simulink model "Attitude_control_RW"  (R2021b)
settings: Solver=VariableStepAuto  StartTime=0.0  StopTime=200  FixedStep=0.0001  RelTol=1e-3
values from neighbouring files (symbols this model uses):
  R = 6378000 + h    (= 7078000)    [dynamicFunctions2.m]
  w0 = sqrt(mu_earth/(R^3))    [dynamicFunctions2.m]
undefined symbols (not defined in the file or in its folder): b, Is, kk, Km, Kt, Q, q_init, Rgyro, Rstr, rw_Inertia, rw_SensorToBody, Ts, unit7, w_dot_init, w_init, wRW_init
libraries: simulink_extras x10, sharedtransform x5, simulink x3, aerolibutil x1, sharedTrackingLibrary x1
settings Model: Creator=sokserey  LastModifiedBy=ASUS
settings SolverCC: ZeroCrossAlgorithm=Adaptive
settings DebuggingCC: IgnoredZcDiagnostic=none

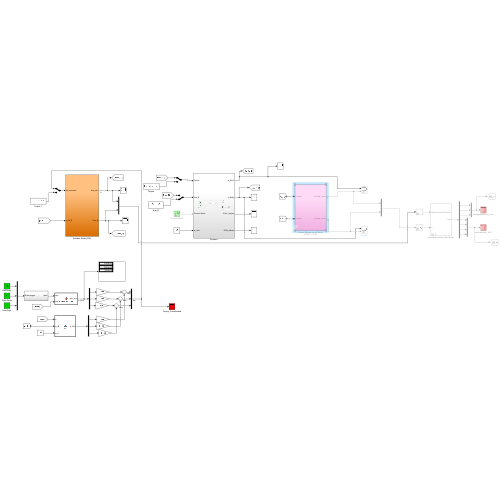
[thumbnail: Simulink's stored preview of the top-level diagram]
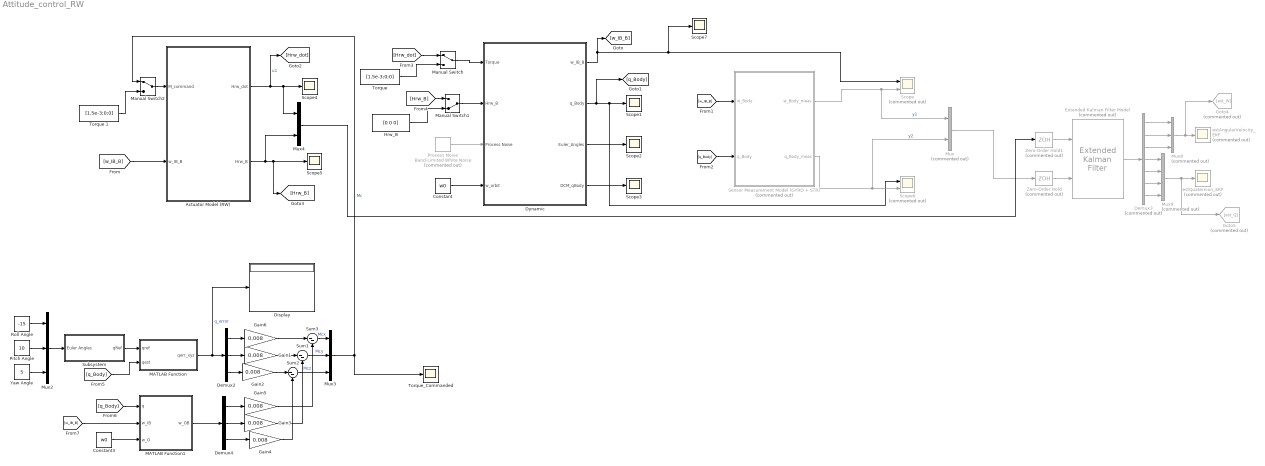
== system Attitude_control_RW ==
  Actuator Model (RW) : Subsystem
  Constant : Constant  Value=w0
  Constant3 : Constant  Value=w0
  Demux2 : Demux  Outputs=3
  Demux3 : Demux  Commented=on  Outputs=7
  Demux4 : Demux  Outputs=3
  Display : Display
  Dynamic : Subsystem
  "Extended Kalman Filter Model " : sharedTrackingLibrary/Extended Kalman Filter  Commented=on  StateTransitionFcn=dynamicFunctions2  HasStateTransitionJacobianFcn=off  HasAdditiveProcessNoise=Additive  ProcessNoise=diag(unit7)*Q  HasTimeVaryingProcessNoise=off  HasStateTransitionFcnExtraArgument=1  InitialState=[w_init; q_init]  InitialStateCovariance=1e-6  MeasurementFcn1=measurementFunction2  HasMeasurementJacobianFcn1=off  HasMeasurementEnablePort1=off  HasAdditiveMeasurementNoise1=Additive  MeasurementNoise1=Rconf4  HasTimeVaryingMeasurementNoise1=off  HasMeasurementFcnExtraArgument1=0  MeasurementFcn2=myMeasurementFcn  HasMeasurementJacobianFcn2=off  HasMeasurementEnablePort2=off  HasAdditiveMeasurementNoise2=Additive  MeasurementNoise2=1  HasTimeVaryingMeasurementNoise2=off  HasMeasurementFcnExtraArgument2=0  MeasurementFcn3=myMeasurementFcn  HasMeasurementJacobianFcn3=off  HasMeasurementEnablePort3=off  HasAdditiveMeasurementNoise3=Additive  MeasurementNoise3=1  HasTimeVaryingMeasurementNoise3=off  HasMeasurementFcnExtraArgument3=0  MeasurementFcn4=myMeasurementFcn  HasMeasurementJacobianFcn4=off  HasMeasurementEnablePort4=off  HasAdditiveMeasurementNoise4=Additive  MeasurementNoise4=1  HasTimeVaryingMeasurementNoise4=off  HasMeasurementFcnExtraArgument4=0  MeasurementFcn5=myMeasurementFcn  HasMeasurementJacobianFcn5=off  HasMeasurementEnablePort5=off  HasAdditiveMeasurementNoise5=Additive  MeasurementNoise5=1  HasTimeVaryingMeasurementNoise5=off  HasMeasurementFcnExtraArgument5=0  EnableMultirate=off  StateTransitionFcnSampleTime=1  MeasurementFcn1SampleTime=1  MeasurementFcn2SampleTime=1  MeasurementFcn3SampleTime=1  MeasurementFcn4SampleTime=1  MeasurementFcn5SampleTime=1  UseCurrentEstimator=on  OutputStateCovariance=off  DataType=double  SampleTime=Ts  NumberOfMeasurements=1
      settings: SourceProductBaseCode=AE,PW,CT,DR,TF,ID,LP,NV,AR,RO,RR,UV,VE
  Gain{1..6} (6 alike) : Gain  Gain=0.008
  Goto4 : Goto  Commented=on  GotoTag=est_W
  Goto5 : Goto  Commented=on  GotoTag=est_Q
  Hrw_B : Constant  Value=[0 0 0]
  MATLAB Function : MATLAB Function  TreatAsAtomicUnit=on
  MATLAB Function1 : MATLAB Function  TreatAsAtomicUnit=on
  Manual Switch : ManualSwitch
  Manual Switch1 : ManualSwitch  CurrentSetting=0
  Manual Switch2 : ManualSwitch
  Mux : Mux  Commented=on  Inputs=2
  Mux2 : Mux  Inputs=3
  Mux3 : Mux  Inputs=3
  Mux4 : Mux  Inputs=2
  Mux8 : Mux  Commented=on  Inputs=3
  Mux9 : Mux  Commented=on
  Pitch Angle : Constant  Value=10
  Process Noise : simulink/Sources/Band-Limited White Noise  Commented=on  Cov=Q*Ts  Ts=Ts  seed=[23341]
  Roll Angle : Constant  Value=-15
  Scope : Scope  Commented=on  NumInputPorts=2
  Scope{1..5,7} (6 alike) : Scope
  Scope6 : Scope  Commented=on  NumInputPorts=2
  Sensor Measurement Model (GYRO + STR) : Subsystem  Commented=on
  Subsystem : Subsystem
  Sum1 : Sum  Inputs=|--
  Sum2 : Sum  Inputs=|--
  Sum3 : Sum  Inputs=|--
  "Torque " : Constant  Value=[1.5e-3;0;0]
  Torque 1 : Constant  Value=[1.5e-3;0;0]
  Torque_Commanded : Scope
  Yaw Angle : Constant  Value=5
  Zero-Order Hold : ZeroOrderHold  Commented=on  SampleTime=Ts
  Zero-Order Hold1 : ZeroOrderHold  Commented=on  SampleTime=Ts
  estAngularVelocity_EKF : Scope  Commented=on
  "estQuaternion_EKF " : Scope  Commented=on
  wires:
  Process Noise/1 -> Dynamic/3("Process Noise ")
  Constant/1 -> Dynamic/4(w_orbit)
  Dynamic/1(w_IB_B) -> [w_IB_B], Scope7/1, Scope/1
  Dynamic/2(q_Body) -> [q_Body], Scope6/1, Scope1/1
  Dynamic/3(Euler_Angles) -> Scope2/1
  Dynamic/4(DCM_qBody) -> Scope3/1
  Zero-Order Hold1/1 -> "Extended Kalman Filter Model "/1
  Demux3/2 -> Mux8/2
  Demux3/3 -> Mux8/3
  Demux3/6 -> Mux9/3
  Demux3/4 -> Mux9/1
  Mux9/1 -> Goto5/1, "estQuaternion_EKF "/1
  Demux3/5 -> Mux9/2
  "Extended Kalman Filter Model "/1 -> Demux3/1
  Demux3/1 -> Mux8/1
  Zero-Order Hold/1 -> "Extended Kalman Filter Model "/2
  [w_IB_B] -> Actuator Model (RW)/2(w_IB_B)
  Actuator Model (RW)/1("Hrw_dot ") -> [Hrw_dot], Mux4/1, Scope4/1  "u1"
  Actuator Model (RW)/2(Hrw_B) -> Mux4/2, [Hrw_B], Scope5/1
  [w_IB_B] -> Sensor Measurement Model (GYRO + STR)/1(w_Body)
  Sensor Measurement Model (GYRO + STR)/1(w_Body_meas) -> Mux/1, Scope/2  "y1"
  [q_Body] -> Sensor Measurement Model (GYRO + STR)/2(q_Body)
  Sensor Measurement Model (GYRO + STR)/2(q_Body_meas) -> Mux/2, Scope6/2  "y2"
  Mux/1 -> Zero-Order Hold/1
  "Torque "/1 -> Manual Switch/2
  Manual Switch1/1 -> Dynamic/2(Hrw_B)
  Hrw_B/1 -> Manual Switch1/2
  [Hrw_dot] -> Manual Switch/1
  [Hrw_B] -> Manual Switch1/1
  Roll Angle/1 -> Mux2/1
  Sum1/1 -> Mux3/2  "Mcy"
  MATLAB Function/1(qerr_xyz) -> Display/1, Demux2/1  "q_error"
  Demux4/2 -> Gain3/1
  Sum3/1 -> Mux3/1  "Mcx"
  Gain2/1 -> Sum2/1
  Sum2/1 -> Mux3/3  "Mcz"
  Demux4/1 -> Gain5/1
  Demux2/2 -> Gain1/1
  Demux2/1 -> Gain6/1
  Gain6/1 -> Sum3/1
  Mux3/1 -> Manual Switch2/1, Torque_Commanded/1  "Mc"
  Yaw Angle/1 -> Mux2/3
  Subsystem/1(qRef) -> MATLAB Function/1(qref)
  Gain1/1 -> Sum1/1
  Pitch Angle/1 -> Mux2/2
  Mux2/1 -> Subsystem/1(Euler Angles)
  Demux2/3 -> Gain2/1
  Mux8/1 -> Goto4/1, estAngularVelocity_EKF/1
  Demux4/3 -> Gain4/1
  Manual Switch2/1 -> Actuator Model (RW)/1("M_command ")
  Torque 1/1 -> Manual Switch2/2
  Demux3/7 -> Mux9/4
  Mux4/1 -> Zero-Order Hold1/1
  [q_Body] -> MATLAB Function/2(qest)
  [q_Body] -> MATLAB Function1/1(q)
  [w_IB_B] -> MATLAB Function1/2(w_IB)
  Constant3/1 -> MATLAB Function1/3(w_O)
  MATLAB Function1/1(w_OB) -> Demux4/1
  Gain5/1 -> Sum3/2
  Gain3/1 -> Sum1/2
  Gain4/1 -> Sum2/2
  Manual Switch/1 -> Dynamic/1(Torque)

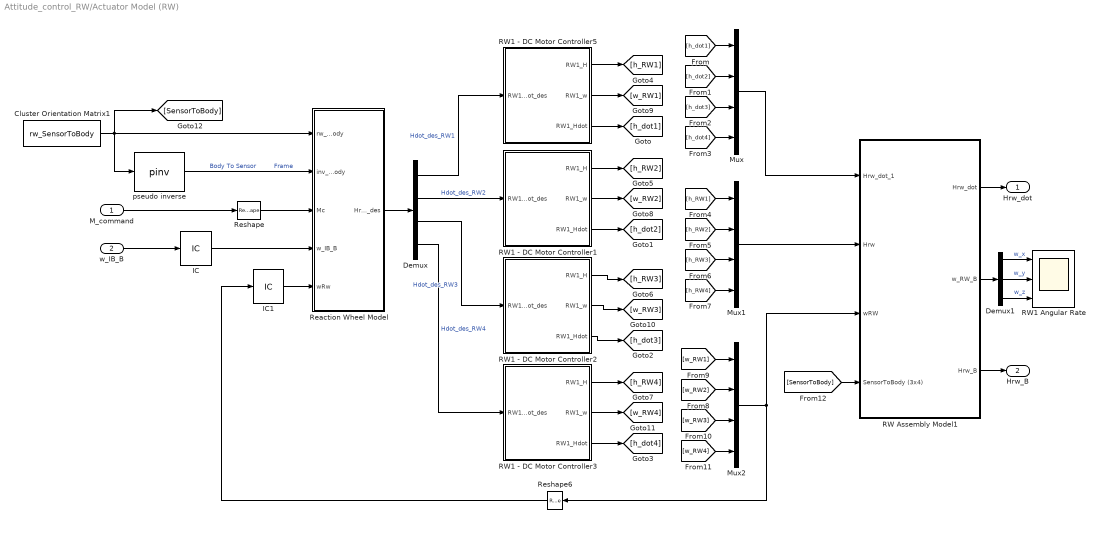
== system Attitude_control_RW/Actuator Model (RW) ==
  "M_command " : Inport
  w_IB_B : Inport  Port=2
  Cluster Orientation Matrix1 : Constant  Value=rw_SensorToBody  VectorParams1D=off  SampleTime=Ts
  Demux : Demux
  Demux1 : Demux  Outputs=3
  IC : InitialCondition  Value=w_init
  IC1 : InitialCondition  Value=wRW_init
  Mux : Mux
  Mux1 : Mux
  Mux2 : Mux
  RW Assembly Model1 : Subsystem
  RW1 - DC Motor Controller1 : Subsystem
  RW1 - DC Motor Controller2 : Subsystem
  RW1 - DC Motor Controller3 : Subsystem
  RW1 - DC Motor Controller5 : Subsystem
  RW1 Angular Rate : Scope  NumInputPorts=3
  Reaction Wheel Model : MATLAB Function  TreatAsAtomicUnit=on
  Reshape : Reshape  OutputDimensionality=Column vector (2-D)
  Reshape6 : Reshape  OutputDimensionality=Column vector (2-D)
  pseudo inverse : MATLABFcn  MATLABFcn=pinv  Output1D=off
  "Hrw_dot " : Outport  VectorParamsAs1DForOutWhenUnconnected=off
  Hrw_B : Outport  Port=2  VectorParamsAs1DForOutWhenUnconnected=off
  wires:
  Demux/1 -> RW1 - DC Motor Controller5/1(RW1_Hdot_des)  "Hdot_des_RW1"
  Demux/2 -> RW1 - DC Motor Controller1/1(RW1_Hdot_des)  "Hdot_des_RW2"
  Demux/3 -> RW1 - DC Motor Controller2/1(RW1_Hdot_des)  "Hdot_des_RW3"
  Demux/4 -> RW1 - DC Motor Controller3/1(RW1_Hdot_des)  "Hdot_des_RW4"
  Demux1/3 -> RW1 Angular Rate/3  "w_z"
  Demux1/1 -> RW1 Angular Rate/1  "w_x"
  Demux1/2 -> RW1 Angular Rate/2  "w_y"
  "M_command "/1 -> Reshape/1
  Reaction Wheel Model/1(Hrw_dot_des) -> Demux/1
  [h_dot1] -> Mux/1
  [h_dot2] -> Mux/2
  [h_dot3] -> Mux/3
  [h_dot4] -> Mux/4
  Mux/1 -> RW Assembly Model1/1(Hrw_dot_1)
  [h_RW1] -> Mux1/1
  [h_RW2] -> Mux1/2
  [h_RW3] -> Mux1/3
  [h_RW4] -> Mux1/4
  Mux1/1 -> RW Assembly Model1/2(Hrw)
  [w_RW2] -> Mux2/2
  [w_RW1] -> Mux2/1
  [w_RW3] -> Mux2/3
  [w_RW4] -> Mux2/4
  pseudo inverse/1 -> Reaction Wheel Model/2(inv_rwSensorToBody)  "Body To Sensor         Frame"
  Reshape/1 -> Reaction Wheel Model/3(Mc)
  Cluster Orientation Matrix1/1 -> pseudo inverse/1, [SensorToBody], Reaction Wheel Model/1(rw_SensorToBody)
  [SensorToBody] -> RW Assembly Model1/4(SensorToBody (3x4))
  RW Assembly Model1/2(w_RW_B) -> Demux1/1
  RW Assembly Model1/1(Hrw_dot) -> "Hrw_dot "/1
  Mux2/1 -> Reshape6/1, RW Assembly Model1/3(wRW)
  Reshape6/1 -> IC1/1
  w_IB_B/1 -> IC/1
  IC/1 -> Reaction Wheel Model/4(w_IB_B)
  IC1/1 -> Reaction Wheel Model/5(wRw)
  RW1 - DC Motor Controller5/2(RW1_w) -> [w_RW1]
  RW1 - DC Motor Controller5/1(RW1_H) -> [h_RW1]
  RW1 - DC Motor Controller5/3(RW1_Hdot) -> [h_dot1]
  RW1 - DC Motor Controller1/1(RW1_H) -> [h_RW2]
  RW1 - DC Motor Controller1/2(RW1_w) -> [w_RW2]
  RW1 - DC Motor Controller1/3(RW1_Hdot) -> [h_dot2]
  RW1 - DC Motor Controller2/1(RW1_H) -> [h_RW3]
  RW1 - DC Motor Controller2/2(RW1_w) -> [w_RW3]
  RW1 - DC Motor Controller2/3(RW1_Hdot) -> [h_dot3]
  RW1 - DC Motor Controller3/1(RW1_H) -> [h_RW4]
  RW1 - DC Motor Controller3/2(RW1_w) -> [w_RW4]
  RW1 - DC Motor Controller3/3(RW1_Hdot) -> [h_dot4]
  RW Assembly Model1/3(Hrw_B) -> Hrw_B/1

== system Attitude_control_RW/Dynamic ==
  Torque : Inport
  Hrw_B : Inport  Port=2
  "Process Noise " : Inport  Port=3
  w_orbit : Inport  Port=4
  Display2 : Display
  Dynamic Model : Subsystem
  Kinematic Model1 : Subsystem
  Subsystem : Subsystem
  Subsystem1 : Subsystem
  Sum1 : Sum  Inputs=|++
  Sum2 : Sum  Inputs=|++
  Terminator : Terminator
  w_IB_B : Outport  VectorParamsAs1DForOutWhenUnconnected=off
  q_Body : Outport  Port=2  VectorParamsAs1DForOutWhenUnconnected=off
  Euler_Angles : Outport  Port=3  VectorParamsAs1DForOutWhenUnconnected=off
  DCM_qBody : Outport  Port=4  VectorParamsAs1DForOutWhenUnconnected=off
  wires:
  Sum2/1 -> Dynamic Model/2("Hrw_B ")
  Dynamic Model/1(w_IB_B) -> Kinematic Model1/1(w_IB_B), w_IB_B/1
  Hrw_B/1 -> Sum2/1
  Sum1/1 -> Dynamic Model/1(Mc+Md)
  Subsystem1/1(Euler Angle) -> Euler_Angles/1
  Torque/1 -> Sum1/1
  Kinematic Model1/2(w_OB_B) -> Terminator/1
  Kinematic Model1/1(qBody) -> Subsystem/1(qest), q_Body/1
  "Process Noise "/1 -> Sum2/2, Sum1/2
  Subsystem/1("DCM ") -> Display2/1, DCM_qBody/1, Subsystem1/1("DCM ")
  w_orbit/1 -> Kinematic Model1/2(w_orbit)

== system Attitude_control_RW/Sensor Measurement Model (GYRO + STR) ==
  w_Body : Inport
  q_Body : Inport  Port=2
  GYRO Sensor Model : Subsystem
  Normalization Model : Subsystem
  Star Tracker Model : Subsystem
  w_Body_meas : Outport  VectorParamsAs1DForOutWhenUnconnected=off
  q_Body_meas : Outport  Port=2  VectorParamsAs1DForOutWhenUnconnected=off
  wires:
  GYRO Sensor Model/1(w_Body_meas) -> w_Body_meas/1
  w_Body/1 -> GYRO Sensor Model/1(w_Body)
  q_Body/1 -> Star Tracker Model/1(q_Body)
  Normalization Model/1(Normalized_u) -> q_Body_meas/1
  Star Tracker Model/1(q_Body_meas) -> Normalization Model/1(u)

== system Attitude_control_RW/Subsystem ==
  Euler Angles : Inport
  Degrees to Radians1 : simulink_extras/Transformations/Degrees to Radians
  Direction Cosine Matrix to Quaternions : sharedtransform/Direction Cosine Matrix  to Quaternions  aMode=0  action=None  tolerance=eps(2)
      settings: SourceProductBaseCode=AE,PW,DR,MT,UV,VE
  Rotation Angles to Direction Cosine Matrix : sharedtransform/Rotation Angles to Direction Cosine Matrix  rotationOrder=ZYX  aMode=aMode
      settings: SourceProductBaseCode=AE,PW,DR,MT,UV,VE
  Subsystem1 : Subsystem
  qRef : Outport  VectorParamsAs1DForOutWhenUnconnected=off
  wires:
  Euler Angles/1 -> Degrees to Radians1/1
  Degrees to Radians1/1 -> Rotation Angles to Direction Cosine Matrix/1
  Rotation Angles to Direction Cosine Matrix/1 -> Direction Cosine Matrix to Quaternions/1
  Direction Cosine Matrix to Quaternions/1 -> Subsystem1/1(q0,q1,q2,q3)
  Subsystem1/1(q1,q2,q3,q4) -> qRef/1

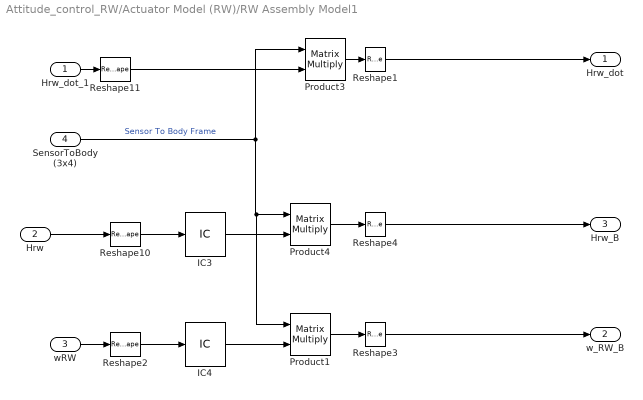
== system Attitude_control_RW/Actuator Model (RW)/RW Assembly Model1 ==
  Hrw_dot_1 : Inport
  Hrw : Inport  Port=2
  wRW : Inport  Port=3
  SensorToBody (3x4) : Inport  Port=4
  IC3 : InitialCondition  Value=[wRW_init(1,1)*rw_Inertia; wRW_init(2,1)*rw_Inertia; wRW_init(3,1)*rw_Inertia;wRW_init(4,1)*rw_Inertia]
  IC4 : InitialCondition  Value=wRW_init
  Product1 : Product  Inputs=**  Multiplication=Matrix(*)  RndMeth=Zero
  Product3 : Product  Inputs=**  Multiplication=Matrix(*)  RndMeth=Zero
  Product4 : Product  Inputs=**  Multiplication=Matrix(*)  RndMeth=Zero
  Reshape{1..4,10..11} (6 alike) : Reshape  OutputDimensionality=Column vector (2-D)
  Hrw_dot : Outport  VectorParamsAs1DForOutWhenUnconnected=off
  w_RW_B : Outport  Port=2  VectorParamsAs1DForOutWhenUnconnected=off
  Hrw_B : Outport  Port=3  VectorParamsAs1DForOutWhenUnconnected=off
  wires:
  SensorToBody (3x4)/1 -> Product3/1, Product1/1, Product4/1  "Sensor To Body Frame"
  Product4/1 -> Reshape4/1
  Reshape1/1 -> Hrw_dot/1
  Reshape4/1 -> Hrw_B/1
  IC3/1 -> Product4/2
  IC4/1 -> Product1/2
  Product1/1 -> Reshape3/1
  Hrw/1 -> Reshape10/1
  Reshape10/1 -> IC3/1
  Reshape2/1 -> IC4/1
  wRW/1 -> Reshape2/1
  Reshape3/1 -> w_RW_B/1
  Reshape11/1 -> Product3/2
  Hrw_dot_1/1 -> Reshape11/1
  Product3/1 -> Reshape1/1

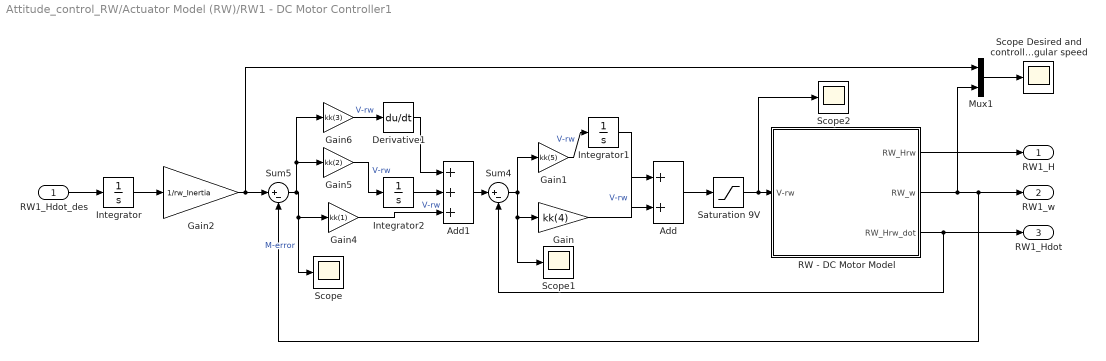
== system Attitude_control_RW/Actuator Model (RW)/RW1 - DC Motor Controller1 ==
  RW1_Hdot_des : Inport
  Add : Sum
  Add1 : Sum  Inputs=+++
  Derivative1 : Derivative
  Gain : Gain  Gain=kk(4)
  Gain1 : Gain  Gain=kk(5)
  Gain2 : Gain  Gain=1/rw_Inertia
  Gain4 : Gain  Gain=kk(1)
  Gain5 : Gain  Gain=kk(2)
  Gain6 : Gain  Gain=kk(3)
  Integrator : Integrator
  Integrator1 : Integrator
  Integrator2 : Integrator
  Mux1 : Mux  Inputs=2
  RW - DC Motor Model : Subsystem
  "Saturation 9V " : Saturate  UpperLimit=9  LowerLimit=-9
  Scope : Scope
  "Scope Desired and controlled RW-angular speed " : Scope
  Scope1 : Scope
  Scope2 : Scope
  Sum4 : Sum  Inputs=|+-
  Sum5 : Sum  Inputs=|+-
  RW1_H : Outport  VectorParamsAs1DForOutWhenUnconnected=off
  RW1_w : Outport  Port=2  VectorParamsAs1DForOutWhenUnconnected=off
  RW1_Hdot : Outport  Port=3  VectorParamsAs1DForOutWhenUnconnected=off
  wires:
  Gain4/1 -> Add1/3  "V-rw"
  Gain6/1 -> Derivative1/1  "V-rw"
  Derivative1/1 -> Add1/1
  RW - DC Motor Model/3(RW_Hrw_dot) -> Sum4/2, RW1_Hdot/1
  Add1/1 -> Sum4/1
  Gain1/1 -> Integrator1/1  "V-rw"
  "Saturation 9V "/1 -> Scope2/1, RW - DC Motor Model/1(V-rw)
  Add/1 -> "Saturation 9V "/1
  Integrator1/1 -> Add/2
  Sum5/1 -> Gain6/1, Gain5/1, Scope/1, Gain4/1  "M-error"
  Mux1/1 -> "Scope Desired and controlled RW-angular speed "/1
  Sum4/1 -> Gain/1, Scope1/1, Gain1/1
  RW - DC Motor Model/1(RW_Hrw) -> RW1_H/1
  Gain5/1 -> Integrator2/1  "V-rw"
  RW1_Hdot_des/1 -> Integrator/1
  RW - DC Motor Model/2(RW_w) -> Sum5/2, RW1_w/1, Mux1/2
  Integrator/1 -> Gain2/1
  Integrator2/1 -> Add1/2
  Gain2/1 -> Mux1/1, Sum5/1
  Gain/1 -> Add/1  "V-rw"

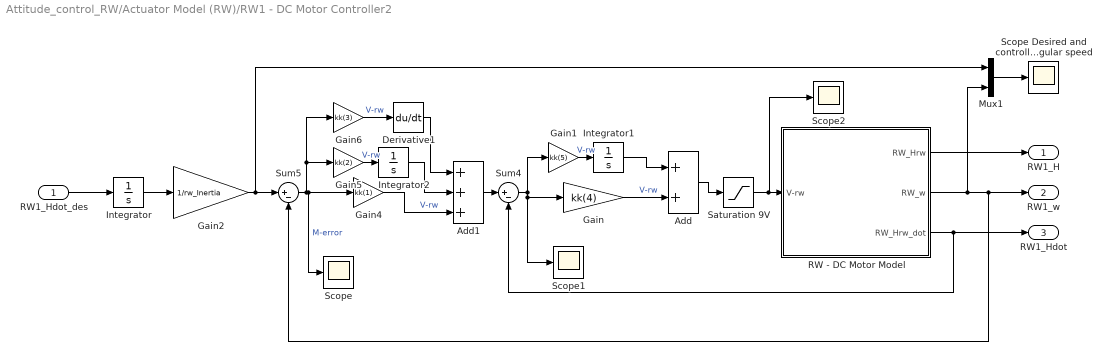
== system Attitude_control_RW/Actuator Model (RW)/RW1 - DC Motor Controller2 ==
  RW1_Hdot_des : Inport
  Add : Sum
  Add1 : Sum  Inputs=+++
  Derivative1 : Derivative
  Gain : Gain  Gain=kk(4)
  Gain1 : Gain  Gain=kk(5)
  Gain2 : Gain  Gain=1/rw_Inertia
  Gain4 : Gain  Gain=kk(1)
  Gain5 : Gain  Gain=kk(2)
  Gain6 : Gain  Gain=kk(3)
  Integrator : Integrator
  Integrator1 : Integrator
  Integrator2 : Integrator
  Mux1 : Mux  Inputs=2
  RW - DC Motor Model : Subsystem
  "Saturation 9V " : Saturate  UpperLimit=9  LowerLimit=-9
  Scope : Scope
  "Scope Desired and controlled RW-angular speed " : Scope
  Scope1 : Scope
  Scope2 : Scope
  Sum4 : Sum  Inputs=|+-
  Sum5 : Sum  Inputs=|+-
  RW1_H : Outport  VectorParamsAs1DForOutWhenUnconnected=off
  RW1_w : Outport  Port=2  VectorParamsAs1DForOutWhenUnconnected=off
  RW1_Hdot : Outport  Port=3  VectorParamsAs1DForOutWhenUnconnected=off
  wires:
  RW1_Hdot_des/1 -> Integrator/1
  Mux1/1 -> "Scope Desired and controlled RW-angular speed "/1
  Integrator2/1 -> Add1/2
  RW - DC Motor Model/2(RW_w) -> RW1_w/1, Sum5/2, Mux1/2
  Integrator/1 -> Gain2/1
  RW - DC Motor Model/1(RW_Hrw) -> RW1_H/1
  Sum5/1 -> Gain6/1, Gain5/1, Scope/1, Gain4/1  "M-error"
  Sum4/1 -> Gain/1, Scope1/1, Gain1/1
  Integrator1/1 -> Add/1
  Gain1/1 -> Integrator1/1  "V-rw"
  Gain5/1 -> Integrator2/1  "V-rw"
  "Saturation 9V "/1 -> Scope2/1, RW - DC Motor Model/1(V-rw)
  Add1/1 -> Sum4/1
  RW - DC Motor Model/3(RW_Hrw_dot) -> Sum4/2, RW1_Hdot/1
  Derivative1/1 -> Add1/1
  Add/1 -> "Saturation 9V "/1
  Gain2/1 -> Mux1/1, Sum5/1
  Gain6/1 -> Derivative1/1  "V-rw"
  Gain4/1 -> Add1/3  "V-rw"
  Gain/1 -> Add/2  "V-rw"

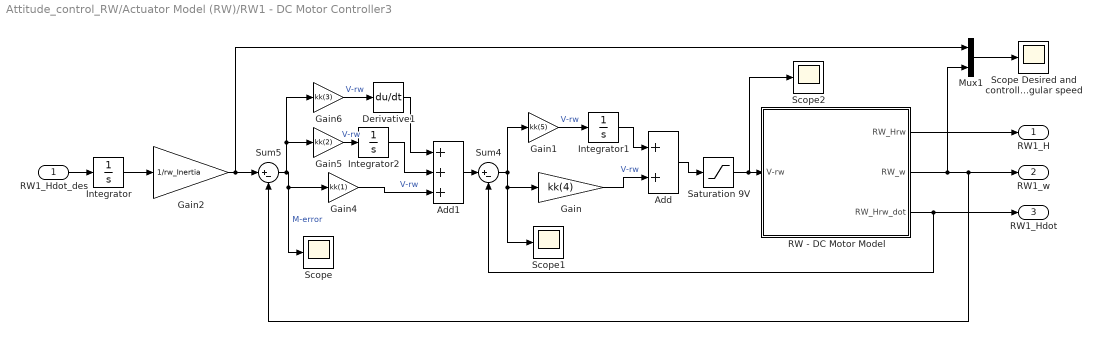
== system Attitude_control_RW/Actuator Model (RW)/RW1 - DC Motor Controller3 ==
  RW1_Hdot_des : Inport
  Add : Sum
  Add1 : Sum  Inputs=+++
  Derivative1 : Derivative
  Gain : Gain  Gain=kk(4)
  Gain1 : Gain  Gain=kk(5)
  Gain2 : Gain  Gain=1/rw_Inertia
  Gain4 : Gain  Gain=kk(1)
  Gain5 : Gain  Gain=kk(2)
  Gain6 : Gain  Gain=kk(3)
  Integrator : Integrator
  Integrator1 : Integrator
  Integrator2 : Integrator
  Mux1 : Mux  Inputs=2
  RW - DC Motor Model : Subsystem
  "Saturation 9V " : Saturate  UpperLimit=9  LowerLimit=-9
  Scope : Scope
  "Scope Desired and controlled RW-angular speed " : Scope
  Scope1 : Scope
  Scope2 : Scope
  Sum4 : Sum  Inputs=|+-
  Sum5 : Sum  Inputs=|+-
  RW1_H : Outport  VectorParamsAs1DForOutWhenUnconnected=off
  RW1_w : Outport  Port=2  VectorParamsAs1DForOutWhenUnconnected=off
  RW1_Hdot : Outport  Port=3  VectorParamsAs1DForOutWhenUnconnected=off
  wires:
  RW1_Hdot_des/1 -> Integrator/1
  Mux1/1 -> "Scope Desired and controlled RW-angular speed "/1
  Integrator2/1 -> Add1/2
  RW - DC Motor Model/2(RW_w) -> RW1_w/1, Sum5/2, Mux1/2
  Integrator/1 -> Gain2/1
  RW - DC Motor Model/1(RW_Hrw) -> RW1_H/1
  Sum5/1 -> Gain6/1, Gain5/1, Scope/1, Gain4/1  "M-error"
  Sum4/1 -> Gain/1, Scope1/1, Gain1/1
  Gain/1 -> Add/2  "V-rw"
  Integrator1/1 -> Add/1
  Gain1/1 -> Integrator1/1  "V-rw"
  Gain5/1 -> Integrator2/1  "V-rw"
  "Saturation 9V "/1 -> Scope2/1, RW - DC Motor Model/1(V-rw)
  Add1/1 -> Sum4/1
  RW - DC Motor Model/3(RW_Hrw_dot) -> Sum4/2, RW1_Hdot/1
  Derivative1/1 -> Add1/1
  Add/1 -> "Saturation 9V "/1
  Gain2/1 -> Mux1/1, Sum5/1
  Gain6/1 -> Derivative1/1  "V-rw"
  Gain4/1 -> Add1/3  "V-rw"

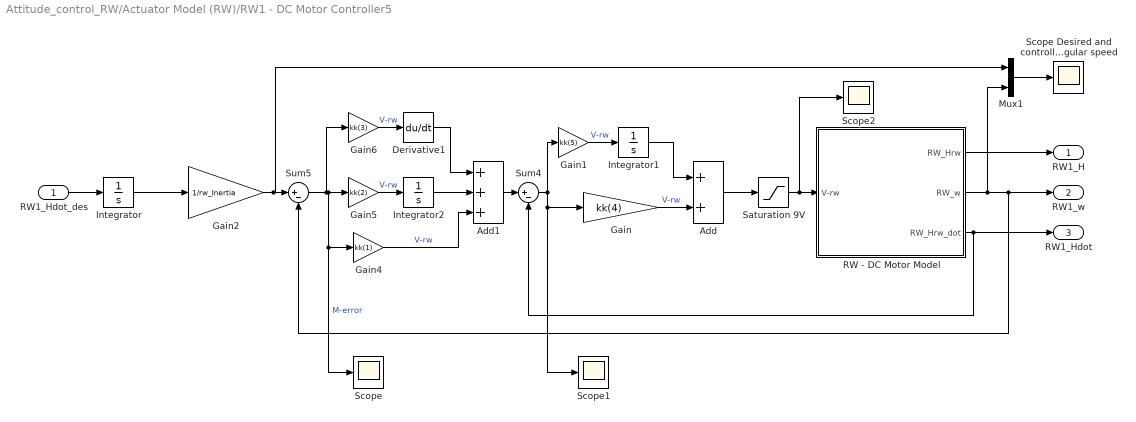
== system Attitude_control_RW/Actuator Model (RW)/RW1 - DC Motor Controller5 ==
  RW1_Hdot_des : Inport
  Add : Sum
  Add1 : Sum  Inputs=+++
  Derivative1 : Derivative
  Gain : Gain  Gain=kk(4)
  Gain1 : Gain  Gain=kk(5)
  Gain2 : Gain  Gain=1/rw_Inertia
  Gain4 : Gain  Gain=kk(1)
  Gain5 : Gain  Gain=kk(2)
  Gain6 : Gain  Gain=kk(3)
  Integrator : Integrator
  Integrator1 : Integrator
  Integrator2 : Integrator
  Mux1 : Mux  Inputs=2
  RW - DC Motor Model : Subsystem
  "Saturation 9V " : Saturate  UpperLimit=9  LowerLimit=-9
  Scope : Scope
  "Scope Desired and controlled RW-angular speed " : Scope
  Scope1 : Scope
  Scope2 : Scope
  Sum4 : Sum  Inputs=|+-
  Sum5 : Sum  Inputs=|+-
  RW1_H : Outport  VectorParamsAs1DForOutWhenUnconnected=off
  RW1_w : Outport  Port=2  VectorParamsAs1DForOutWhenUnconnected=off
  RW1_Hdot : Outport  Port=3  VectorParamsAs1DForOutWhenUnconnected=off
  wires:
  Integrator/1 -> Gain2/1
  RW1_Hdot_des/1 -> Integrator/1
  RW - DC Motor Model/1(RW_Hrw) -> RW1_H/1
  Sum4/1 -> Gain1/1, Scope1/1, Gain/1
  RW - DC Motor Model/2(RW_w) -> Sum5/2, RW1_w/1, Mux1/2
  Add1/1 -> Sum4/1
  Sum5/1 -> Gain5/1, Scope/1, Gain4/1, Gain6/1  "M-error"
  Mux1/1 -> "Scope Desired and controlled RW-angular speed "/1
  Gain2/1 -> Mux1/1, Sum5/1
  "Saturation 9V "/1 -> Scope2/1, RW - DC Motor Model/1(V-rw)
  RW - DC Motor Model/3(RW_Hrw_dot) -> Sum4/2, RW1_Hdot/1
  Add/1 -> "Saturation 9V "/1
  Gain1/1 -> Integrator1/1  "V-rw"
  Gain/1 -> Add/2  "V-rw"
  Integrator1/1 -> Add/1
  Derivative1/1 -> Add1/1
  Gain6/1 -> Derivative1/1  "V-rw"
  Integrator2/1 -> Add1/2
  Gain4/1 -> Add1/3  "V-rw"
  Gain5/1 -> Integrator2/1  "V-rw"

== system Attitude_control_RW/Dynamic/Dynamic Model ==
  Mc+Md : Inport
  "Hrw_B " : Inport  Port=2
  Add : Sum  Inputs=-+
  Add1 : Sum
  Constant1 : Constant  Value=Is
  Embedded MATLAB Function : MATLAB Function  TreatAsAtomicUnit=on
  IC : InitialCondition  Value=w_init
  IC1 : InitialCondition  Value=w_dot_init
  Integrator : Integrator  InitialConditionSource=external  InitialCondition=[0;0;0]
  Invert 3x3 Matrix : aerolibutil/Invert  3x3 Matrix
  Product : Product  Multiplication=Matrix(*)  RndMeth=Zero
  Product1 : Product  Multiplication=Matrix(*)  RndMeth=Zero
  Reshape : Reshape  OutputDimensionality=Column vector (2-D)
  Reshape1 : Reshape  OutputDimensionality=Column vector (2-D)
  w_initial : Constant  Value=w_init  VectorParams1D=off  SampleTime=-1
  w_IB_B : Outport  VectorParamsAs1DForOutWhenUnconnected=off
  wires:
  Constant1/1 -> Invert 3x3 Matrix/1, Product/1
  IC/1 -> Product/2, Embedded MATLAB Function/1(w)
  Mc+Md/1 -> Reshape1/1
  Invert 3x3 Matrix/1 -> Product1/1
  Integrator/1 -> w_IB_B/1, IC/1
  Product1/1 -> IC1/1
  Embedded MATLAB Function/1(y) -> Reshape/1
  w_initial/1 -> Integrator/2
  Add/1 -> Product1/2
  IC1/1 -> Integrator/1
  Reshape/1 -> Add/1
  Reshape1/1 -> Add/2
  Product/1 -> Add1/1
  Add1/1 -> Embedded MATLAB Function/2(Iw_plus_hwheel)
  "Hrw_B "/1 -> Add1/2

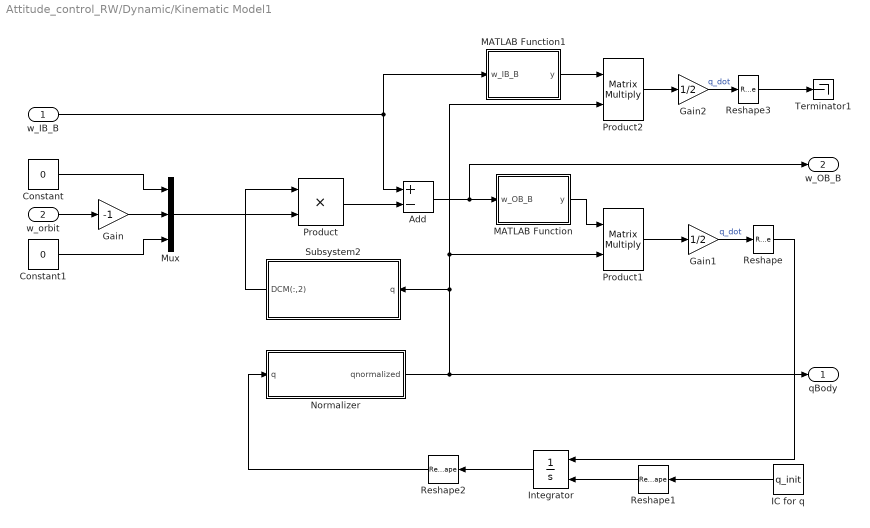
== system Attitude_control_RW/Dynamic/Kinematic Model1 ==
  w_IB_B : Inport
  w_orbit : Inport  Port=2
  Add : Sum  Inputs=+-
  Constant : Constant  Value=0
  Constant1 : Constant  Value=0
  Gain : Gain  Gain=-1
  Gain1 : Gain  Gain=1/2
  Gain2 : Gain  Gain=1/2
  IC for q : Constant  Value=q_init  SampleTime=Ts
  Integrator : Integrator  InitialConditionSource=external
  MATLAB Function : MATLAB Function  TreatAsAtomicUnit=on
  MATLAB Function1 : MATLAB Function  TreatAsAtomicUnit=on
  Mux : Mux  Inputs=3
  Normalizer : MATLAB Function  TreatAsAtomicUnit=on
  Product : Product
  Product1 : Product  Multiplication=Matrix(*)
  Product2 : Product  Multiplication=Matrix(*)
  Reshape{,1..3} (4 alike) : Reshape  OutputDimensionality=Column vector (2-D)
  Subsystem2 : Subsystem
  Terminator1 : Terminator
  qBody : Outport  VectorParamsAs1DForOutWhenUnconnected=off
  w_OB_B : Outport  Port=2  VectorParamsAs1DForOutWhenUnconnected=off
  wires:
  Reshape2/1 -> Normalizer/1(q)
  Product/1 -> Add/2
  Integrator/1 -> Reshape2/1
  Normalizer/1(qnormalized) -> qBody/1, Subsystem2/1(q), Product1/2, Product2/2
  IC for q/1 -> Reshape1/1
  Reshape1/1 -> Integrator/2
  Add/1 -> MATLAB Function/1(w_OB_B), w_OB_B/1
  w_orbit/1 -> Gain/1
  Mux/1 -> Product/2
  Constant/1 -> Mux/1
  Constant1/1 -> Mux/3
  Product1/1 -> Gain1/1
  MATLAB Function/1(y) -> Product1/1
  Gain1/1 -> Reshape/1  "q_dot"
  w_IB_B/1 -> MATLAB Function1/1(w_IB_B), Add/1
  Product2/1 -> Gain2/1
  MATLAB Function1/1(y) -> Product2/1
  Gain2/1 -> Reshape3/1  "q_dot"
  Subsystem2/1(DCM(:,2)) -> Product/1
  Gain/1 -> Mux/2
  Reshape/1 -> Integrator/1
  Reshape3/1 -> Terminator1/1

== system Attitude_control_RW/Dynamic/Subsystem ==
  qest : Inport
  Quaternions to Direction Cosine Matrix : sharedtransform/Quaternions to  Direction Cosine Matrix  aMode=aMode
      settings: SourceProductBaseCode=AE,PW,DR,MT,UV,VE
  Subsystem : Subsystem
  "DCM " : Outport  VectorParamsAs1DForOutWhenUnconnected=off
  wires:
  Quaternions to Direction Cosine Matrix/1 -> "DCM "/1
  Subsystem/1(q0,q1,q2,q3) -> Quaternions to Direction Cosine Matrix/1
  qest/1 -> Subsystem/1(q1,q2,q3,q4)

== system Attitude_control_RW/Dynamic/Subsystem1 ==
  "DCM " : Inport
  Direction Cosine Matrix to Rotation Angles : sharedtransform/Direction Cosine Matrix to Rotation Angles  rotationOrder=ZYX  aMode=aMode  action=None  tolerance=eps(2)
      settings: SourceProductBaseCode=AE,PW,DR,MT,UV,VE
  Radians to Degrees1 : simulink_extras/Transformations/Radians to Degrees
  Euler Angle : Outport  VectorParamsAs1DForOutWhenUnconnected=off
  wires:
  Radians to Degrees1/1 -> Euler Angle/1
  Direction Cosine Matrix to Rotation Angles/1 -> Radians to Degrees1/1
  "DCM "/1 -> Direction Cosine Matrix to Rotation Angles/1

== system Attitude_control_RW/Sensor Measurement Model (GYRO + STR)/GYRO Sensor Model ==
  w_Body : Inport
  Gyroscope Model : Subsystem
  Zero-Order Hold2 : ZeroOrderHold  SampleTime=Ts
  w_Body_meas : Outport  VectorParamsAs1DForOutWhenUnconnected=off
  wires:
  w_Body/1 -> Gyroscope Model/1(w_Body)
  Gyroscope Model/1(Gyro1_wmeas) -> Zero-Order Hold2/1
  Zero-Order Hold2/1 -> w_Body_meas/1

== system Attitude_control_RW/Sensor Measurement Model (GYRO + STR)/Normalization Model ==
  u : Inport
  Divide : Product  Inputs=*/
  MATLAB Function : MATLAB Function  TreatAsAtomicUnit=on
  Math Function2 : Math  Operator=square  SignedPower=on  SaturateOnIntegerOverflow=on
  Sum of Elements : Sum  Inputs=+
  Normalized_u : Outport  VectorParamsAs1DForOutWhenUnconnected=off
  wires:
  Divide/1 -> Normalized_u/1
  MATLAB Function/1(y) -> Divide/2
  Sum of Elements/1 -> MATLAB Function/1(u)
  u/1 -> Divide/1, Math Function2/1
  Math Function2/1 -> Sum of Elements/1

== system Attitude_control_RW/Sensor Measurement Model (GYRO + STR)/Star Tracker Model ==
  q_Body : Inport
  Scope : Scope
  StarTracker 1 Error Model3 : Subsystem  TreatAsAtomicUnit=on
  Zero-Order Hold2 : ZeroOrderHold  SampleTime=0.1
  q_Body_meas : Outport  VectorParamsAs1DForOutWhenUnconnected=off
  wires:
  Zero-Order Hold2/1 -> Scope/1, q_Body_meas/1
  q_Body/1 -> StarTracker 1 Error Model3/1("q_Body ")
  StarTracker 1 Error Model3/1("q_body_meas ") -> Zero-Order Hold2/1

== system Attitude_control_RW/Subsystem/Subsystem1 ==
  q0,q1,q2,q3 : Inport
  Demux1 : Demux
  Mux1 : Mux
  q1,q2,q3,q4 : Outport  VectorParamsAs1DForOutWhenUnconnected=off
  wires:
  q0,q1,q2,q3/1 -> Demux1/1
  Mux1/1 -> q1,q2,q3,q4/1
  Demux1/1 -> Mux1/4
  Demux1/2 -> Mux1/1
  Demux1/3 -> Mux1/2
  Demux1/4 -> Mux1/3

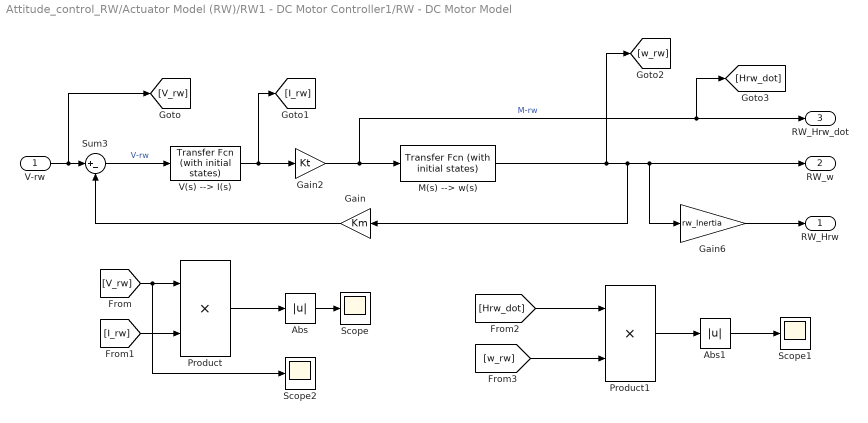
== system Attitude_control_RW/Actuator Model (RW)/RW1 - DC Motor Controller1/RW - DC Motor Model ==
  V-rw : Inport
  Abs : Abs
  Abs1 : Abs
  Gain : Gain  Gain=Km
  Gain2 : Gain  Gain=Kt
  Gain6 : Gain  Gain=rw_Inertia
  M(s) --> w(s) : simulink_extras/Additional Linear/Transfer Fcn (with initial states)  N=[1]  D=[5e-4 b]  X0=0
  Product : Product
  Product1 : Product
  Scope : Scope
  Scope1 : Scope
  Scope2 : Scope
  Sum3 : Sum  Inputs=|+-
  V(s) --> I(s) : simulink_extras/Additional Linear/Transfer Fcn (with initial states)  N=1  D=[R]  X0=0
  RW_Hrw : Outport  VectorParamsAs1DForOutWhenUnconnected=off
  RW_w : Outport  Port=2  VectorParamsAs1DForOutWhenUnconnected=off
  RW_Hrw_dot : Outport  Port=3  VectorParamsAs1DForOutWhenUnconnected=off
  wires:
  V-rw/1 -> [V_rw], Sum3/1
  Gain2/1 -> M(s) --> w(s)/1, [Hrw_dot], RW_Hrw_dot/1  "M-rw"
  Gain6/1 -> RW_Hrw/1
  Gain/1 -> Sum3/2
  Sum3/1 -> V(s) --> I(s)/1  "V-rw"
  V(s) --> I(s)/1 -> [I_rw], Gain2/1
  M(s) --> w(s)/1 -> RW_w/1, Gain6/1, Gain/1, [w_rw]
  [V_rw] -> Scope2/1, Product/1
  [I_rw] -> Product/2
  Product/1 -> Abs/1
  Abs/1 -> Scope/1
  [Hrw_dot] -> Product1/1
  [w_rw] -> Product1/2
  Product1/1 -> Abs1/1
  Abs1/1 -> Scope1/1

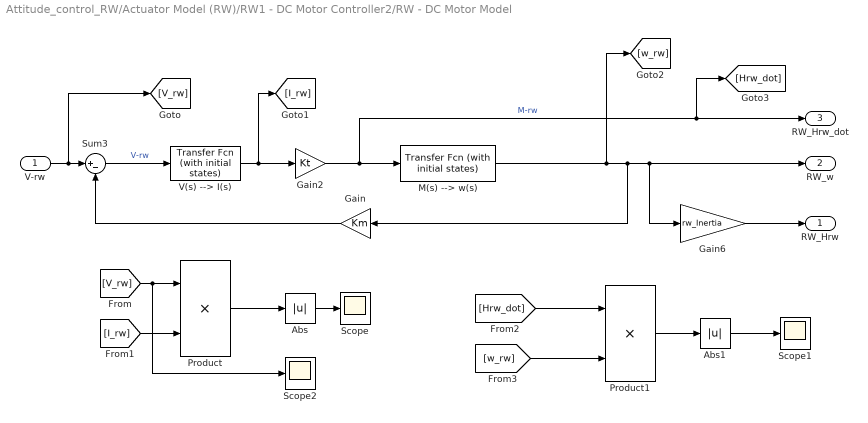
== system Attitude_control_RW/Actuator Model (RW)/RW1 - DC Motor Controller2/RW - DC Motor Model ==
  V-rw : Inport
  Abs : Abs
  Abs1 : Abs
  Gain : Gain  Gain=Km
  Gain2 : Gain  Gain=Kt
  Gain6 : Gain  Gain=rw_Inertia
  M(s) --> w(s) : simulink_extras/Additional Linear/Transfer Fcn (with initial states)  N=[1]  D=[5e-4 b]  X0=0
  Product : Product
  Product1 : Product
  Scope : Scope
  Scope1 : Scope
  Scope2 : Scope
  Sum3 : Sum  Inputs=|+-
  V(s) --> I(s) : simulink_extras/Additional Linear/Transfer Fcn (with initial states)  N=1  D=[R]  X0=0
  RW_Hrw : Outport  VectorParamsAs1DForOutWhenUnconnected=off
  RW_w : Outport  Port=2  VectorParamsAs1DForOutWhenUnconnected=off
  RW_Hrw_dot : Outport  Port=3  VectorParamsAs1DForOutWhenUnconnected=off
  wires:
  V-rw/1 -> [V_rw], Sum3/1
  Gain2/1 -> M(s) --> w(s)/1, [Hrw_dot], RW_Hrw_dot/1  "M-rw"
  Gain6/1 -> RW_Hrw/1
  Gain/1 -> Sum3/2
  Sum3/1 -> V(s) --> I(s)/1  "V-rw"
  V(s) --> I(s)/1 -> [I_rw], Gain2/1
  M(s) --> w(s)/1 -> RW_w/1, Gain6/1, Gain/1, [w_rw]
  [V_rw] -> Scope2/1, Product/1
  [I_rw] -> Product/2
  Product/1 -> Abs/1
  Abs/1 -> Scope/1
  [Hrw_dot] -> Product1/1
  [w_rw] -> Product1/2
  Product1/1 -> Abs1/1
  Abs1/1 -> Scope1/1

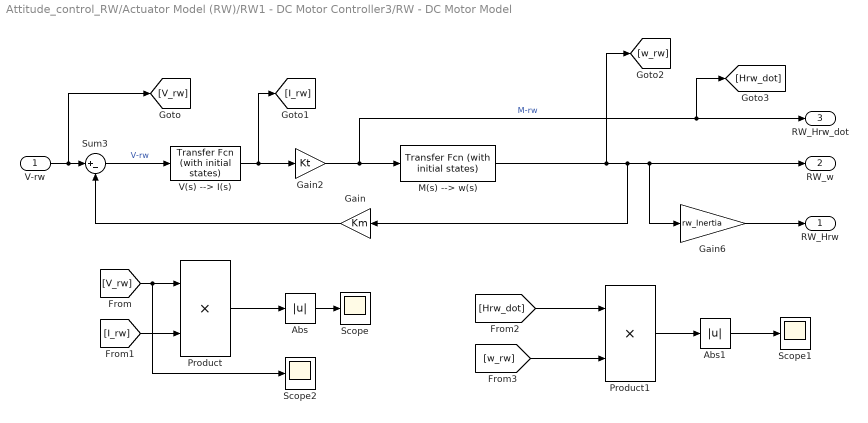
== system Attitude_control_RW/Actuator Model (RW)/RW1 - DC Motor Controller3/RW - DC Motor Model ==
  V-rw : Inport
  Abs : Abs
  Abs1 : Abs
  Gain : Gain  Gain=Km
  Gain2 : Gain  Gain=Kt
  Gain6 : Gain  Gain=rw_Inertia
  M(s) --> w(s) : simulink_extras/Additional Linear/Transfer Fcn (with initial states)  N=[1]  D=[5e-4 b]  X0=0
  Product : Product
  Product1 : Product
  Scope : Scope
  Scope1 : Scope
  Scope2 : Scope
  Sum3 : Sum  Inputs=|+-
  V(s) --> I(s) : simulink_extras/Additional Linear/Transfer Fcn (with initial states)  N=1  D=[R]  X0=0
  RW_Hrw : Outport  VectorParamsAs1DForOutWhenUnconnected=off
  RW_w : Outport  Port=2  VectorParamsAs1DForOutWhenUnconnected=off
  RW_Hrw_dot : Outport  Port=3  VectorParamsAs1DForOutWhenUnconnected=off
  wires:
  V-rw/1 -> [V_rw], Sum3/1
  Gain2/1 -> M(s) --> w(s)/1, [Hrw_dot], RW_Hrw_dot/1  "M-rw"
  Gain6/1 -> RW_Hrw/1
  Gain/1 -> Sum3/2
  Sum3/1 -> V(s) --> I(s)/1  "V-rw"
  V(s) --> I(s)/1 -> [I_rw], Gain2/1
  M(s) --> w(s)/1 -> RW_w/1, Gain6/1, Gain/1, [w_rw]
  [V_rw] -> Scope2/1, Product/1
  [I_rw] -> Product/2
  Product/1 -> Abs/1
  Abs/1 -> Scope/1
  [Hrw_dot] -> Product1/1
  [w_rw] -> Product1/2
  Product1/1 -> Abs1/1
  Abs1/1 -> Scope1/1

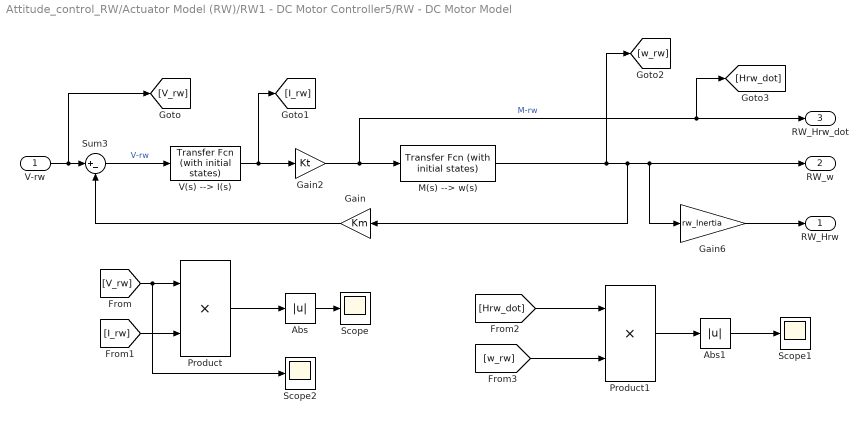
== system Attitude_control_RW/Actuator Model (RW)/RW1 - DC Motor Controller5/RW - DC Motor Model ==
  V-rw : Inport
  Abs : Abs
  Abs1 : Abs
  Gain : Gain  Gain=Km
  Gain2 : Gain  Gain=Kt
  Gain6 : Gain  Gain=rw_Inertia
  M(s) --> w(s) : simulink_extras/Additional Linear/Transfer Fcn (with initial states)  N=[1]  D=[5e-4 b]  X0=0
  Product : Product
  Product1 : Product
  Scope : Scope
  Scope1 : Scope
  Scope2 : Scope
  Sum3 : Sum  Inputs=|+-
  V(s) --> I(s) : simulink_extras/Additional Linear/Transfer Fcn (with initial states)  N=1  D=[R]  X0=0
  RW_Hrw : Outport  VectorParamsAs1DForOutWhenUnconnected=off
  RW_w : Outport  Port=2  VectorParamsAs1DForOutWhenUnconnected=off
  RW_Hrw_dot : Outport  Port=3  VectorParamsAs1DForOutWhenUnconnected=off
  wires:
  V-rw/1 -> [V_rw], Sum3/1
  Gain2/1 -> M(s) --> w(s)/1, [Hrw_dot], RW_Hrw_dot/1  "M-rw"
  Gain6/1 -> RW_Hrw/1
  Gain/1 -> Sum3/2
  Sum3/1 -> V(s) --> I(s)/1  "V-rw"
  V(s) --> I(s)/1 -> [I_rw], Gain2/1
  M(s) --> w(s)/1 -> RW_w/1, Gain6/1, Gain/1, [w_rw]
  [V_rw] -> Scope2/1, Product/1
  [I_rw] -> Product/2
  Product/1 -> Abs/1
  Abs/1 -> Scope/1
  [Hrw_dot] -> Product1/1
  [w_rw] -> Product1/2
  Product1/1 -> Abs1/1
  Abs1/1 -> Scope1/1

== system Attitude_control_RW/Dynamic/Kinematic Model1/Subsystem2 ==
  q : Inport
  MATLAB Function : MATLAB Function  TreatAsAtomicUnit=on
  Quaternions to Direction Cosine Matrix : sharedtransform/Quaternions to  Direction Cosine Matrix  aMode=aMode
      settings: SourceProductBaseCode=AE,PW,DR,MT,UV,VE
  Reshape2 : Reshape  OutputDimensionality=Column vector (2-D)
  Subsystem : Subsystem
  DCM(:,2) : Outport  VectorParamsAs1DForOutWhenUnconnected=off
  wires:
  Subsystem/1(q0,q1,q2,q3) -> Quaternions to Direction Cosine Matrix/1
  q/1 -> Subsystem/1(q1,q2,q3,q4)
  Quaternions to Direction Cosine Matrix/1 -> MATLAB Function/1(DCM)
  MATLAB Function/1(DCM_2) -> Reshape2/1
  Reshape2/1 -> DCM(:,2)/1

== system Attitude_control_RW/Dynamic/Subsystem/Subsystem ==
  q1,q2,q3,q4 : Inport
  Demux1 : Demux
  Mux1 : Mux
  q0,q1,q2,q3 : Outport  VectorParamsAs1DForOutWhenUnconnected=off
  wires:
  Demux1/2 -> Mux1/3
  q1,q2,q3,q4/1 -> Demux1/1
  Mux1/1 -> q0,q1,q2,q3/1
  Demux1/4 -> Mux1/1
  Demux1/1 -> Mux1/2
  Demux1/3 -> Mux1/4

== system Attitude_control_RW/Sensor Measurement Model (GYRO + STR)/GYRO Sensor Model/Gyroscope Model ==
  w_Body : Inport
  Add : Sum
  Band-Limited White Noise : simulink/Sources/Band-Limited White Noise  Cov=Rgyro*Ts  Ts=Ts  seed=[23341]
  Saturation1 : Saturate  UpperLimit=abs(1000)  LowerLimit=-abs(1000)
  Gyro1_wmeas : Outport  VectorParamsAs1DForOutWhenUnconnected=off
  wires:
  Add/1 -> Saturation1/1
  Saturation1/1 -> Gyro1_wmeas/1
  w_Body/1 -> Add/1
  Band-Limited White Noise/1 -> Add/2

== system Attitude_control_RW/Sensor Measurement Model (GYRO + STR)/Star Tracker Model/StarTracker 1 Error Model3 ==
  "q_Body " : Inport
  Add : Sum
  Band-Limited White Noise : simulink/Sources/Band-Limited White Noise  Cov=Rstr*Ts  Ts=Ts  seed=[12345]
  "q_body_meas " : Outport  VectorParamsAs1DForOutWhenUnconnected=off
  wires:
  Band-Limited White Noise/1 -> Add/2
  "q_Body "/1 -> Add/1
  Add/1 -> "q_body_meas "/1

== system Attitude_control_RW/Dynamic/Kinematic Model1/Subsystem2/Subsystem ==
  q1,q2,q3,q4 : Inport
  Demux1 : Demux
  Mux1 : Mux
  q0,q1,q2,q3 : Outport  VectorParamsAs1DForOutWhenUnconnected=off
  wires:
  Demux1/2 -> Mux1/3
  q1,q2,q3,q4/1 -> Demux1/1
  Mux1/1 -> q0,q1,q2,q3/1
  Demux1/4 -> Mux1/1
  Demux1/1 -> Mux1/2
  Demux1/3 -> Mux1/4

== matlab function Attitude_control_RW/MATLAB Function1 ==
  data: q input; w_OB output; w_IB input; w_O input
function w_OB = fcn(q,w_IB,w_O)

w_OB = [w_IB(1)+2*(q(1)*q(2)+q(3)*q(4))*w_O;
        w_IB(2)+(q(4)^2-q(1)^2+q(2)^2-q(3)^2)*w_O;
        w_IB(3)+2*(q(2)*q(3)-q(1)*q(4))*w_O];

== matlab function Attitude_control_RW/Dynamic/Dynamic Model/Embedded MATLAB Function ==
  data: w input; y output; Iw_plus_hwheel input
function y = crossproduct(w,Iw_plus_hwheel)
% This block supports the Embedded MATLAB subset.
% See the help menu for details. 

%Just used to calculate the cross-product of two inputs
y = cross(w,Iw_plus_hwheel);

== matlab function Attitude_control_RW/Dynamic/Kinematic Model1/Subsystem2/MATLAB Function ==
  data: DCM input; DCM_2 output
function DCM_2 = fcn(DCM)
DCM_2 = DCM(:,2);
end

== matlab function Attitude_control_RW/Dynamic/Kinematic Model1/MATLAB Function ==
  data: w_OB_B input; y output
function y = skew_wOB_B(w_OB_B)


y = [0, w_OB_B(3,1), -w_OB_B(2,1), w_OB_B(1,1);...
    -w_OB_B(3,1), 0, w_OB_B(1,1), w_OB_B(2,1);...
     w_OB_B(2,1), -w_OB_B(1,1), 0, w_OB_B(3,1);...
    -w_OB_B(1,1), -w_OB_B(2,1), -w_OB_B(3,1), 0];
end

== matlab function Attitude_control_RW/Dynamic/Kinematic Model1/Normalizer ==
  data: qnormalized output; q input
function qnormalized = fcn(q)

%Normalizes the quaternion

qnormalized = q;
qs = q(4);
qv = [q(1); q(2); q(3)];

qnormalized(4)= qs /norm(q);
qnormalized(1)= qv(1)/norm(q);
qnormalized(2)= qv(2)/norm(q);
qnormalized(3)= qv(3)/norm(q);

== matlab function Attitude_control_RW/Dynamic/Kinematic Model1/MATLAB Function1 ==
  data: w_IB_B input; y output
function y = skew_wIB_B(w_IB_B)


y = [0, w_IB_B(3,1), -w_IB_B(2,1), w_IB_B(1,1);...
    -w_IB_B(3,1), 0, w_IB_B(1,1), w_IB_B(2,1);...
     w_IB_B(2,1), -w_IB_B(1,1), 0, w_IB_B(3,1);...
    -w_IB_B(1,1), -w_IB_B(2,1), -w_IB_B(3,1), 0];
end

== matlab function Attitude_control_RW/Actuator Model (RW)/Reaction Wheel Model ==
  data: rw_SensorToBody input; Hrw_dot_des output; inv_rwSensorToBody input; Mc input; w_IB_B input; wRw input
function Hrw_dot_des = rwModel(rw_SensorToBody,inv_rwSensorToBody,Mc,w_IB_B,wRw)
% The desired torque is calculated for each reaction wheel 

% The required momentum input
% wRw               (4x1) matrix
% rwInertia_matrix  (4x4) matrix
% rw_SensorToBody   (3x4) matrix
rwInertia = 5e-4; % RW moment of inertia (kg-m2)
rwInertia_matrix = eye(4,4)* rwInertia;
Hrw = rwInertia_matrix * wRw; 

% Hrw_B     (3x1) matrix
% Hrw_B_dot (3x1) matrix
% From Actuator Frame to Satellite Body Frame
Hrw_B = rw_SensorToBody * Hrw ;

% Desired reaction wheel torque in Body Frame
Hrw_B_dot = -Mc - cross(w_IB_B,Hrw_B) ;

% Desired reaction wheel torque in Actuator Frame
Hrw_dot_des = inv_rwSensorToBody * Hrw_B_dot ; 

end

== matlab function Attitude_control_RW/MATLAB Function ==
  data: qref input; qerr_xyz output; qest input
function qerr_xyz  = quaternionError(qref, qest)

qerr = [qest(4)  qest(3) -qest(2) qest(1);...
       -qest(3)  qest(4)  qest(1) qest(2);...
        qest(2) -qest(1)  qest(4) qest(3);...
       -qest(1) -qest(2) -qest(3) qest(4)]*[-qref(1);-qref(2);-qref(3);qref(4)]; % Verify

qerr_xyz = [qerr(1,1); qerr(2,1); qerr(3,1)];   
qerr_4 = qerr(4,1);
qerr_xyz = qerr_xyz*qerr_4;
% qerr_x = qerr(1,1);
% qerr_y = qerr(2,1);
% qerr_z = qerr(3,1);
%qerr_4 = qerr(4,1);
%qerr_xyz*qerr_4;

end
% % 
% function qerr_xyz  = quaternionError(qref, qest)
% 
% qerr = [qref(4)  -qref(3) qref(2) qref(1);...
%         qref(3)  qref(4)  -qref(1) qref(2);...
%         -qref(2) qref(1)  qref(4) qref(3);...
%        -qref(1) -qref(2) -qref(3) qref(4)]*[-qest(1);-qest(2);-qest(3);qest(4)];
% 
% qerr_xyz = [qerr(1,1); qerr(2,1); qerr(3,1)];     
% % qerr_x = qerr(1,1);
% % qerr_y = qerr(2,1);
% % qerr_z = qerr(3,1);
% 
% end

== matlab function Attitude_control_RW/Sensor Measurement Model (GYRO + STR)/Normalization Model/MATLAB Function ==
  data: u input; y output
function y = Sqrt(u)
%#codegen

y = sqrt(u);
